simulink model "Helicopter_SetPoints"  (R2018a)
settings: Solver=VariableStepAuto  StartTime=0.0  StopTime=inf  RelTol=1e-3
values from neighbouring files (symbols this model uses):
  Ad = sys_d.a    [Helicopter_Values.m]
  Bd = sys_d.b    [Helicopter_Values.m]
  Bp = 0.01    [Helicopter_Values.m]
  By = 0.08    [Helicopter_Values.m]
  Cd = sys_d.c    [Helicopter_Values.m]
  g = 9.81    [Helicopter_Values.m]
  jeqp = 0.0172    [Helicopter_Values.m]
  jeqy = 0.021    [Helicopter_Values.m]
  kpp = 0.0556    [Helicopter_Values.m]
  kpy = 0.005    [Helicopter_Values.m]
  kyp = 0.15    [Helicopter_Values.m]
  kyy = 0.21084    [Helicopter_Values.m]
  lcm = 0.015    [Helicopter_Values.m]
  mheli = 0.479    [Helicopter_Values.m]
  p_r_op = -10*pi/180    (= -0.174532925199)    [Helicopter_Values.m]
  Vmp_op = (kyy*mheli*g*cos(p_r_op)*lcm)/(kyy*kpp -kyp*kpy)    [Helicopter_Values.m]
  Vmy_op = kyp*Vmp_op/kyy    [Helicopter_Values.m]
  wp_op = 0    [Helicopter_Values.m]
  wy_op = 0    [Helicopter_Values.m]
  y_r_op = pi/2    (= 1.57079632679)    [Helicopter_Values.m]
undefined symbols (not defined in the file or in its folder): K, k_lqr
libraries: realtime_pacer_lib x1
settings Model: Creator=pacoa  LastModifiedBy=pacoa

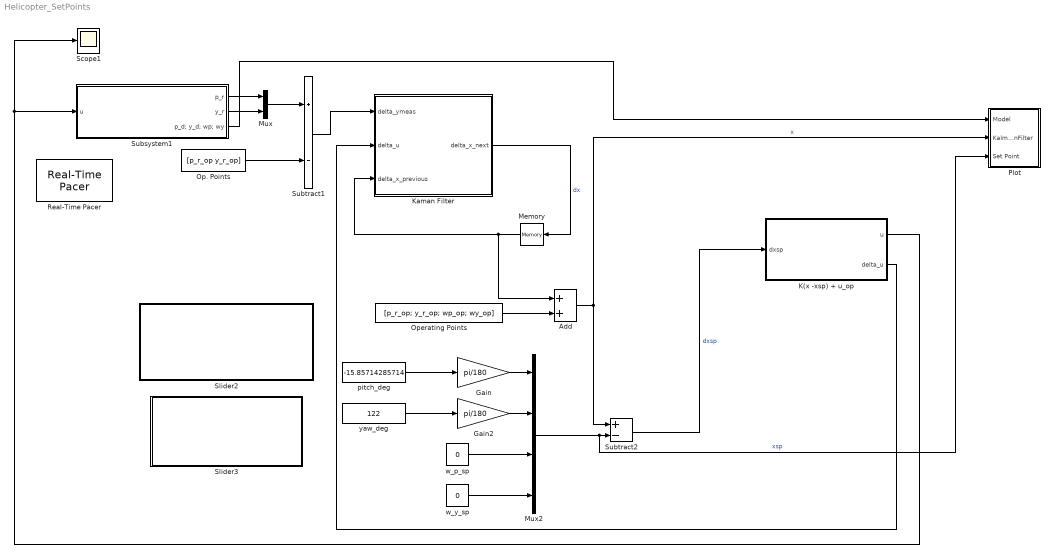
== system Helicopter_SetPoints ==
  Add : Sum
  Gain : Gain  Gain=pi/180
  Gain2 : Gain  Gain=pi/180
  "K(x -xsp) + u_op " : Subsystem
  Kaman Filter : MATLAB Function  TreatAsAtomicUnit=on
  Memory : Memory  InitialCondition=[0;0;0;0]
  Mux : Mux  Inputs=2
  Mux2 : Mux
  Op. Points : Constant  Value=[p_r_op y_r_op]
  Operating Points : Constant  Value=[p_r_op; y_r_op; wp_op; wy_op]
  Plot : Subsystem
  Real-Time Pacer : realtime_pacer_lib/Real-Time Pacer  simTimePerRealTime=10
  Scope1 : Scope
  Slider2 : Subsystem  DialogController=hmiCreateDDGDialog  IsWebBlock=on  mask(MWDashboardBlock){webBlockId=4346c81c-e5d4-41da-88ba-4ceee90b391b, webBlockType=slider, ShowInLibBrowser=on, ShowInitialText=on, HMISrcModelName=Helicopter_SetPoints}
      mask prompts: webBlockId "WebBlock Id"; webBlockType "WebBlock Type"; HMISrcModelName "Source Model"
      mask help: SimulinkHMI:dialogs:SliderDialogDesc
      mask Help: helpview([docroot '/mapfiles/simulink.map'], 'hmi_slider')
      mask Display:
      | if strcmp(get_param(bdroot(gcb),'BlockDiagramType'), 'library')
      |     image([(matlabroot) '/toolbox/simulink/hmi/icons/Slider.png']);
      | end
  Slider3 : Subsystem  DialogController=hmiCreateDDGDialog  IsWebBlock=on  mask(MWDashboardBlock){webBlockId=44ebcc4a-aa43-4d83-9862-a30861b04c6c, webBlockType=slider, ShowInLibBrowser=on, ShowInitialText=on, HMISrcModelName=Helicopter_SetPoints}
      mask prompts: webBlockId "WebBlock Id"; webBlockType "WebBlock Type"; HMISrcModelName "Source Model"
      mask help: SimulinkHMI:dialogs:SliderDialogDesc
      mask Help: helpview([docroot '/mapfiles/simulink.map'], 'hmi_slider')
      mask Display:
      | if strcmp(get_param(bdroot(gcb),'BlockDiagramType'), 'library')
      |     image([(matlabroot) '/toolbox/simulink/hmi/icons/Slider.png']);
      | end
  Subsystem1 : Subsystem
  Subtract1 : Sum  Inputs=+-
  Subtract2 : Sum  Inputs=+-
  pitch_deg : Constant  Value=-15.85714285714
  w_p_sp : Constant  Value=0
  w_y_sp : Constant  Value=0
  yaw_deg : Constant  Value=122
  wires:
  Operating Points/1 -> Add/2
  w_p_sp/1 -> Mux2/3
  Gain2/1 -> Mux2/2
  Gain/1 -> Mux2/1
  Mux2/1 -> Plot/3(Set Point), Subtract2/2  "xsp"
  Kaman Filter/1(delta_x_next) -> Memory/1  "dx"
  Memory/1 -> Kaman Filter/3(delta_x_previous), Add/1
  Subsystem1/2(y_r) -> Mux/2
  Subsystem1/3(p_d; y_d; wp; wy) -> Plot/1(Model)
  Op. Points/1 -> Subtract1/2
  Subsystem1/1(p_r) -> Mux/1
  w_y_sp/1 -> Mux2/4
  Add/1 -> Plot/2(KalmanFilter), Subtract2/1  "x"
  Subtract1/1 -> Kaman Filter/1(delta_ymeas)
  Mux/1 -> Subtract1/1
  Subtract2/1 -> "K(x -xsp) + u_op "/1(dxsp)  "dxsp"
  "K(x -xsp) + u_op "/1(u) -> Subsystem1/1(u), Scope1/1
  "K(x -xsp) + u_op "/2(delta_u) -> Kaman Filter/2(delta_u)
  yaw_deg/1 -> Gain2/1
  pitch_deg/1 -> Gain/1

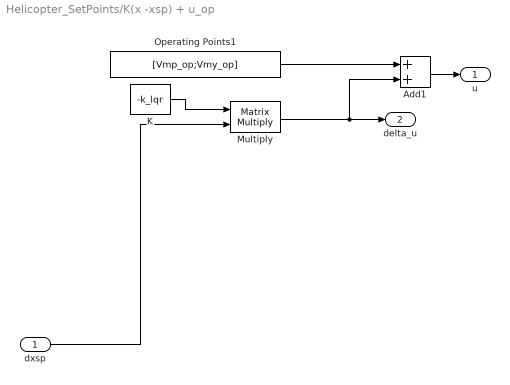
== system Helicopter_SetPoints/K(x -xsp) + u_op  ==
  dxsp : Inport
  Add1 : Sum
  K : Constant  Value=-k_lqr
  Multiply : Product  Multiplication=Matrix(*)
  Operating Points1 : Constant  Value=[Vmp_op;Vmy_op]
  u : Outport
  delta_u : Outport  Port=2
  wires:
  Multiply/1 -> delta_u/1, Add1/2
  Operating Points1/1 -> Add1/1
  dxsp/1 -> Multiply/2
  K/1 -> Multiply/1
  Add1/1 -> u/1

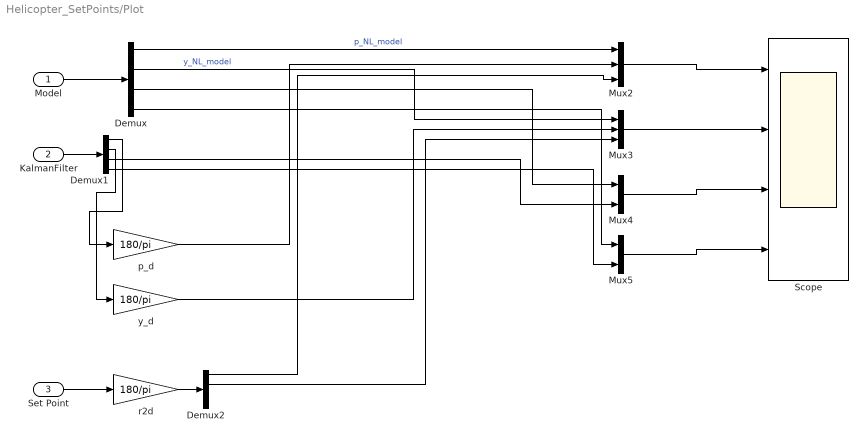
== system Helicopter_SetPoints/Plot ==
  Model : Inport
  KalmanFilter : Inport  Port=2
  Set Point : Inport  Port=3
  Demux : Demux
  Demux1 : Demux
  Demux2 : Demux
  Mux2 : Mux  Inputs=3
  Mux3 : Mux  Inputs=3
  Mux4 : Mux  Inputs=2
  Mux5 : Mux  Inputs=2
  Scope : Scope  NumInputPorts=4
  p_d : Gain  Gain=180/pi
  r2d : Gain  Gain=180/pi
  y_d : Gain  Gain=180/pi
  wires:
  KalmanFilter/1 -> Demux1/1
  Mux2/1 -> Scope/1
  Demux/3 -> Mux4/1
  Demux1/4 -> Mux5/2
  Mux4/1 -> Scope/3
  Demux1/3 -> Mux4/2
  Demux/1 -> Mux2/1  "p_NL_model"
  Demux/4 -> Mux5/1
  Mux3/1 -> Scope/2
  p_d/1 -> Mux2/2
  Mux5/1 -> Scope/4
  Demux1/1 -> p_d/1
  y_d/1 -> Mux3/2
  Demux/2 -> Mux3/1  "y_NL_model"
  Demux1/2 -> y_d/1
  Model/1 -> Demux/1
  Set Point/1 -> r2d/1
  r2d/1 -> Demux2/1
  Demux2/1 -> Mux2/3
  Demux2/2 -> Mux3/3

== system Helicopter_SetPoints/Slider2 ==

== system Helicopter_SetPoints/Slider3 ==

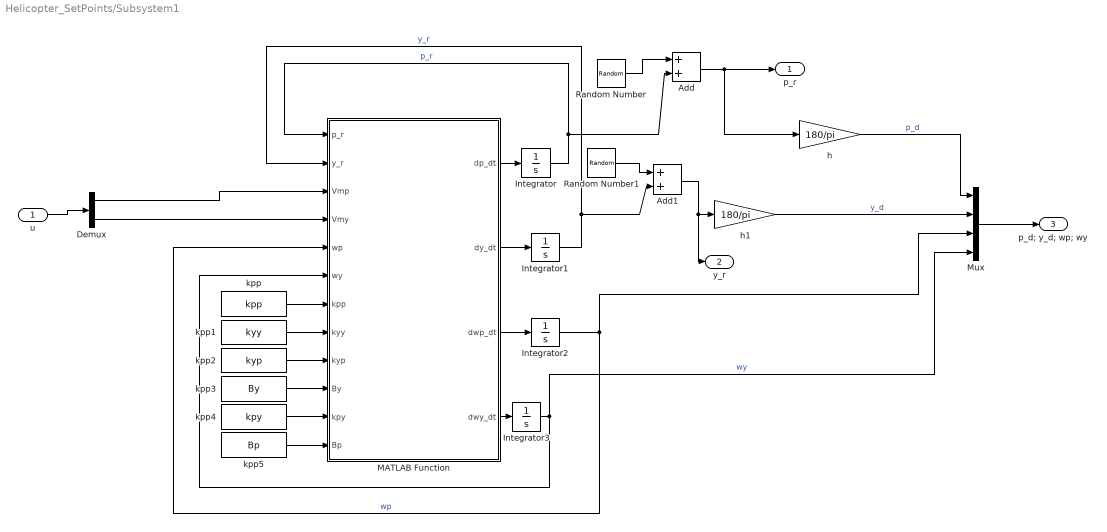
== system Helicopter_SetPoints/Subsystem1 ==
  u : Inport
  Add : Sum
  Add1 : Sum
  Demux : Demux  Outputs=2
  Integrator : Integrator  InitialCondition=(p_r_op)  LimitOutput=on  UpperSaturationLimit=pi/4  LowerSaturationLimit=-pi/4
  Integrator1 : Integrator  InitialCondition=(y_r_op)  LimitOutput=on  UpperSaturationLimit=pi  LowerSaturationLimit=0
  Integrator2 : Integrator  UpperSaturationLimit=1  LowerSaturationLimit=-1
  Integrator3 : Integrator
  MATLAB Function : MATLAB Function  TreatAsAtomicUnit=on
  Mux : Mux
  Random Number : RandomNumber  Variance=0.0005  SampleTime=0.1
  Random Number1 : RandomNumber  Variance=0.0005  SampleTime=0.1
  h : Gain  Gain=180/pi
  h1 : Gain  Gain=180/pi
  kpp : Constant  Value=kpp
  kpp1 : Constant  Value=kyy
  kpp2 : Constant  Value=kyp
  kpp3 : Constant  Value=By
  kpp4 : Constant  Value=kpy
  kpp5 : Constant  Value=Bp
  p_r : Outport  PortDimensions=1
  y_r : Outport  Port=2  PortDimensions=1
  p_d; y_d; wp; wy : Outport  Port=3  PortDimensions=[4 1]
  wires:
  kpp/1 -> MATLAB Function/7(kpp)
  Demux/2 -> MATLAB Function/4(Vmy)
  kpp2/1 -> MATLAB Function/9(kyp)
  kpp4/1 -> MATLAB Function/11(kpy)
  MATLAB Function/3(dwp_dt) -> Integrator2/1
  Integrator1/1 -> Add1/2, MATLAB Function/2(y_r)  "y_r"
  Integrator3/1 -> Mux/4, MATLAB Function/6(wy)  "wy"
  MATLAB Function/1(dp_dt) -> Integrator/1
  h/1 -> Mux/1  "p_d"
  kpp3/1 -> MATLAB Function/10(By)
  kpp1/1 -> MATLAB Function/8(kyy)
  MATLAB Function/4(dwy_dt) -> Integrator3/1
  Integrator/1 -> Add/2, MATLAB Function/1(p_r)  "p_r"
  h1/1 -> Mux/2  "y_d"
  Integrator2/1 -> Mux/3, MATLAB Function/5(wp)  "wp"
  MATLAB Function/2(dy_dt) -> Integrator1/1
  kpp5/1 -> MATLAB Function/12(Bp)
  Mux/1 -> p_d; y_d; wp; wy/1
  Demux/1 -> MATLAB Function/3(Vmp)
  Random Number/1 -> Add/1
  Add/1 -> h/1, p_r/1
  Random Number1/1 -> Add1/1
  Add1/1 -> y_r/1, h1/1
  u/1 -> Demux/1

== matlab function Helicopter_SetPoints/Kaman Filter ==
  data: delta_ymeas input size=[2 1]; delta_u input size=[2 1]; delta_x_next output size=[4 1]; delta_x_previous input size=[4 1]; K parameter size=[4 2]; Ad parameter; Bd parameter; Cd parameter size=[2 4]
function delta_x_next = mykalman(delta_ymeas,delta_u,delta_x_previous, K, Ad, Bd, Cd)

delta_x_next = Ad*delta_x_previous +Bd*delta_u +K*(delta_ymeas -Cd*delta_x_previous);

== matlab function Helicopter_SetPoints/Subsystem1/MATLAB Function ==
  data: p_r input; y_r input; Vmp input; Vmy input; wp input; dp_dt output size=[1 1]; wy input; dy_dt output size=[1 1]; dwp_dt output size=[1 1]; dwy_dt output size=[1 1]; lcm parameter; mheli parameter; jeqp parameter; jeqy parameter; g parameter; kpp input; kyy input; kyp input; By input; kpy input; Bp input
function [dp_dt, dy_dt, dwp_dt, dwy_dt]= fcn(p_r,y_r,Vmp, Vmy,wp,wy, lcm, mheli, jeqp, jeqy, g, kpp, kyy, kyp, By, kpy, Bp)

  %%Parameters
%   
%   Bp,
%   By,
%   g,
%   kpp,
%   kyp,
%   kyy,
%   kpy,
%   mheli,
%   lcm,
%   jeqp,
%   jeqy,
  

%%
   dp_dt = wp;
   dy_dt = wy;
   
   %%
   dwp_dt_n1 = (kpp*Vmp);
   dwp_dt_n2 = (kpy*Vmy);
   dwp_dt_n3 = (Bp*wp+ (mheli*(wy.^2)*sin(p_r)*(lcm^2)*cos(p_r) + (mheli*g*cos(p_r)*lcm)));
   
   dwp_dt_d = (jeqp + mheli*(lcm^2));
   
   dwp_dt = (dwp_dt_n1 -dwp_dt_n2 - dwp_dt_n3)/(dwp_dt_d);
   
   %%
   dwy_dt_n1 = kyp*Vmp;
   dwy_dt_n2 = kyy*Vmy;
   dwy_dt_n3 = 2*mheli*(wy)*sin(p_r)*(lcm^2)*cos(p_r)*wp;
   dwy_dt_n4 = By*wy;
   
   dwy_dt_d = jeqy + mheli*((cos(p_r))^2)*(lcm^2);
   
   dwy_dt = (dwy_dt_n1 - dwy_dt_n2 + dwy_dt_n3 -dwy_dt_n4)/(dwy_dt_d);
